simulink model "SingleTrack"  (Simulink 10.3)
settings: Solver=ode45  StartTime=0.0  StopTime=inf  FixedStep=0.001  RelTol=1e-3
PreLoadFcn:
  | SingleTrack_params
undefined symbols (not defined in the file or in its folder): Car_Bdy1_mass, Car_Steering_i, Car_Whl_Radius, Car_WhlBaseF, Car_WhlBaseR, mEngineMax, PT_DL_iDiff, PT_GearBox_iForwardGears
libraries: CarMaker4SL x9
(part 4 of 4)

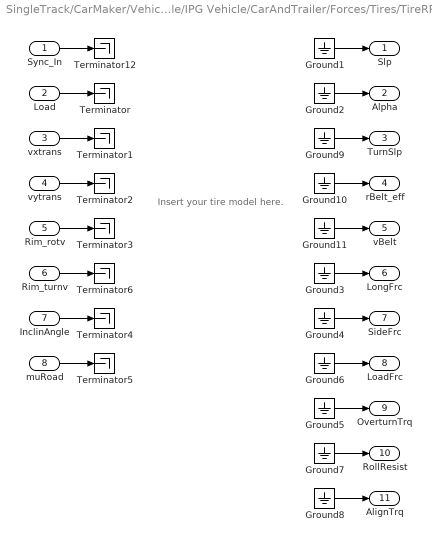
== system SingleTrack/CarMaker/Vehicle/IPG Vehicle/CarAndTrailer/Forces/Tires/TireRR ==
  note: Insert your tire model here.
  Sync_In : Inport
  Load : Inport  Port=2
  vxtrans : Inport  Port=3
  vytrans : Inport  Port=4
  Rim_rotv : Inport  Port=5
  Rim_turnv : Inport  Port=6
  InclinAngle : Inport  Port=7
  muRoad : Inport  Port=8
  Ground{1..11} (11 alike) : Ground
  Terminator{,1..6,12} (8 alike) : Terminator
  Slp : Outport  VectorParamsAs1DForOutWhenUnconnected=off
  Alpha : Outport  Port=2  VectorParamsAs1DForOutWhenUnconnected=off
  TurnSlp : Outport  Port=3  VectorParamsAs1DForOutWhenUnconnected=off
  rBelt_eff : Outport  Port=4  VectorParamsAs1DForOutWhenUnconnected=off
  vBelt : Outport  Port=5  VectorParamsAs1DForOutWhenUnconnected=off
  LongFrc : Outport  Port=6  VectorParamsAs1DForOutWhenUnconnected=off
  SideFrc : Outport  Port=7  VectorParamsAs1DForOutWhenUnconnected=off
  LoadFrc : Outport  Port=8  VectorParamsAs1DForOutWhenUnconnected=off
  OverturnTrq : Outport  Port=9  VectorParamsAs1DForOutWhenUnconnected=off
  RollResist : Outport  Port=10  VectorParamsAs1DForOutWhenUnconnected=off
  AlignTrq : Outport  Port=11  VectorParamsAs1DForOutWhenUnconnected=off
  wires:
  Ground11/1 -> vBelt/1
  Ground10/1 -> rBelt_eff/1
  Ground9/1 -> TurnSlp/1
  Rim_turnv/1 -> Terminator6/1
  Sync_In/1 -> Terminator12/1
  Ground2/1 -> Alpha/1
  Ground3/1 -> LongFrc/1
  Ground4/1 -> SideFrc/1
  Ground5/1 -> OverturnTrq/1
  vxtrans/1 -> Terminator1/1
  vytrans/1 -> Terminator2/1
  Rim_rotv/1 -> Terminator3/1
  InclinAngle/1 -> Terminator4/1
  muRoad/1 -> Terminator5/1
  Load/1 -> Terminator/1
  Ground1/1 -> Slp/1
  Ground6/1 -> LoadFrc/1
  Ground7/1 -> RollResist/1
  Ground8/1 -> AlignTrq/1

== system SingleTrack/CarMaker/Vehicle/User Vehicle (CM4SL)/CarAndTrailer/CreateBus Vhcl.Fr1/Tr2Fr0/Subsystem_00 ==
  sincos : Inport
  Bus Selector : BusSelector  OutputSignals=cry,crz
  Product : Product  RndMeth=Zero
  Tr2Fr1_00 : Outport  VectorParamsAs1DForOutWhenUnconnected=off
  wires:
  sincos/1 -> Bus Selector/1
  Product/1 -> Tr2Fr1_00/1
  Bus Selector/1 -> Product/1  "<cry>"
  Bus Selector/2 -> Product/2  "<crz>"

== system SingleTrack/CarMaker/Vehicle/User Vehicle (CM4SL)/CarAndTrailer/CreateBus Vhcl.Fr1/Tr2Fr0/Subsystem_01 ==
  sincos : Inport
  Add : Sum  Inputs=+-
  Bus Selector : BusSelector  OutputSignals=srx,sry,crz,crx,srz
  Product : Product  Inputs=3  RndMeth=Zero
  Product1 : Product  RndMeth=Zero
  Tr2Fr1_01 : Outport  VectorParamsAs1DForOutWhenUnconnected=off
  wires:
  sincos/1 -> Bus Selector/1
  Product/1 -> Add/1
  Product1/1 -> Add/2
  Add/1 -> Tr2Fr1_01/1
  Bus Selector/1 -> Product/1  "<srx>"
  Bus Selector/2 -> Product/2  "<sry>"
  Bus Selector/3 -> Product/3  "<crz>"
  Bus Selector/4 -> Product1/1  "<crx>"
  Bus Selector/5 -> Product1/2  "<srz>"

== system SingleTrack/CarMaker/Vehicle/User Vehicle (CM4SL)/CarAndTrailer/CreateBus Vhcl.Fr1/Tr2Fr0/Subsystem_02 ==
  sincos : Inport
  Add : Sum
  Bus Selector : BusSelector  OutputSignals=crx,sry,crz,srx,srz
  Product : Product  Inputs=3  RndMeth=Zero
  Product1 : Product  RndMeth=Zero
  Tr2Fr1_02 : Outport  VectorParamsAs1DForOutWhenUnconnected=off
  wires:
  Add/1 -> Tr2Fr1_02/1
  Product1/1 -> Add/2
  Product/1 -> Add/1
  sincos/1 -> Bus Selector/1
  Bus Selector/1 -> Product/1  "<crx>"
  Bus Selector/2 -> Product/2  "<sry>"
  Bus Selector/3 -> Product/3  "<crz>"
  Bus Selector/5 -> Product1/2  "<srz>"
  Bus Selector/4 -> Product1/1  "<srx>"

== system SingleTrack/CarMaker/Vehicle/User Vehicle (CM4SL)/CarAndTrailer/CreateBus Vhcl.Fr1/Tr2Fr0/Subsystem_10 ==
  sincos : Inport
  Bus Selector : BusSelector  OutputSignals=cry,srz
  Product : Product  RndMeth=Zero
  Tr2Fr1_10 : Outport  VectorParamsAs1DForOutWhenUnconnected=off
  wires:
  Bus Selector/2 -> Product/2  "<srz>"
  Bus Selector/1 -> Product/1  "<cry>"
  Product/1 -> Tr2Fr1_10/1
  sincos/1 -> Bus Selector/1

== system SingleTrack/CarMaker/Vehicle/User Vehicle (CM4SL)/CarAndTrailer/CreateBus Vhcl.Fr1/Tr2Fr0/Subsystem_11 ==
  sincos : Inport
  Add : Sum
  Bus Selector : BusSelector  OutputSignals=srx,sry,srz,crx,crz
  Product : Product  Inputs=3  RndMeth=Zero
  Product1 : Product  RndMeth=Zero
  Tr2Fr1_11 : Outport  VectorParamsAs1DForOutWhenUnconnected=off
  wires:
  sincos/1 -> Bus Selector/1
  Product/1 -> Add/1
  Product1/1 -> Add/2
  Add/1 -> Tr2Fr1_11/1
  Bus Selector/1 -> Product/1  "<srx>"
  Bus Selector/2 -> Product/2  "<sry>"
  Bus Selector/3 -> Product/3  "<srz>"
  Bus Selector/5 -> Product1/2  "<crz>"
  Bus Selector/4 -> Product1/1  "<crx>"

== system SingleTrack/CarMaker/Vehicle/User Vehicle (CM4SL)/CarAndTrailer/CreateBus Vhcl.Fr1/Tr2Fr0/Subsystem_12 ==
  sincos : Inport
  Add : Sum  Inputs=+-
  Bus Selector : BusSelector  OutputSignals=crx,sry,srz,srx,crz
  Product : Product  Inputs=3  RndMeth=Zero
  Product1 : Product  RndMeth=Zero
  Tr2Fr1_12 : Outport  VectorParamsAs1DForOutWhenUnconnected=off
  wires:
  Add/1 -> Tr2Fr1_12/1
  Product1/1 -> Add/2
  Product/1 -> Add/1
  sincos/1 -> Bus Selector/1
  Bus Selector/1 -> Product/1  "<crx>"
  Bus Selector/2 -> Product/2  "<sry>"
  Bus Selector/3 -> Product/3  "<srz>"
  Bus Selector/5 -> Product1/2  "<crz>"
  Bus Selector/4 -> Product1/1  "<srx>"

== system SingleTrack/CarMaker/Vehicle/User Vehicle (CM4SL)/CarAndTrailer/CreateBus Vhcl.Fr1/Tr2Fr0/Subsystem_20 ==
  sincos : Inport
  Bus Selector : BusSelector  OutputSignals=sry
  Gain : Gain  Gain=-1
  Tr2Fr1_20 : Outport  VectorParamsAs1DForOutWhenUnconnected=off
  wires:
  sincos/1 -> Bus Selector/1
  Gain/1 -> Tr2Fr1_20/1
  Bus Selector/1 -> Gain/1  "<sry>"

== system SingleTrack/CarMaker/Vehicle/User Vehicle (CM4SL)/CarAndTrailer/CreateBus Vhcl.Fr1/Tr2Fr0/Subsystem_21 ==
  sincos : Inport
  Bus Selector : BusSelector  OutputSignals=srx,cry
  Product : Product  RndMeth=Zero
  Tr2Fr1_21 : Outport  VectorParamsAs1DForOutWhenUnconnected=off
  wires:
  sincos/1 -> Bus Selector/1
  Product/1 -> Tr2Fr1_21/1
  Bus Selector/1 -> Product/1  "<srx>"
  Bus Selector/2 -> Product/2  "<cry>"

== system SingleTrack/CarMaker/Vehicle/User Vehicle (CM4SL)/CarAndTrailer/CreateBus Vhcl.Fr1/Tr2Fr0/Subsystem_22 ==
  sincos : Inport
  Bus Selector : BusSelector  OutputSignals=crx,cry
  Product : Product  RndMeth=Zero
  Tr2Fr1_22 : Outport  VectorParamsAs1DForOutWhenUnconnected=off
  wires:
  Product/1 -> Tr2Fr1_22/1
  sincos/1 -> Bus Selector/1
  Bus Selector/1 -> Product/1  "<crx>"
  Bus Selector/2 -> Product/2  "<cry>"

== system SingleTrack/CarMaker/Vehicle/User Vehicle (CM4SL)/CarAndTrailer/CreateBus Vhcl.Fr1/Tr2Fr0/sincos ==
  Car : Inport
  Bus Creator : BusCreator  Inputs=6
  Bus Selector : BusSelector  OutputSignals=Road_Fr1_rx,Road_Fr1_ry,Car_Yaw
  Trigonometric Function : Trigonometry
  Trigonometric Function1 : Trigonometry  Operator=cos
  Trigonometric Function2 : Trigonometry
  Trigonometric Function3 : Trigonometry
  Trigonometric Function4 : Trigonometry  Operator=cos
  Trigonometric Function5 : Trigonometry  Operator=cos
  sincos : Outport  VectorParamsAs1DForOutWhenUnconnected=off
  wires:
  Bus Selector/1 -> Trigonometric Function/1, Trigonometric Function1/1  "<Road_Fr1_rx>"
  Bus Selector/2 -> Trigonometric Function3/1, Trigonometric Function4/1  "<Road_Fr1_ry>"
  Bus Selector/3 -> Trigonometric Function2/1, Trigonometric Function5/1  "<Car_Yaw>"
  Car/1 -> Bus Selector/1
  Trigonometric Function5/1 -> Bus Creator/6  "crz"
  Trigonometric Function4/1 -> Bus Creator/5  "cry"
  Trigonometric Function1/1 -> Bus Creator/4  "crx"
  Trigonometric Function2/1 -> Bus Creator/3  "srz"
  Trigonometric Function3/1 -> Bus Creator/2  "sry"
  Trigonometric Function/1 -> Bus Creator/1  "srx"
  Bus Creator/1 -> sincos/1

== system SingleTrack/CarMaker/Vehicle/User Vehicle (CM4SL)/CarAndTrailer/PowerTrainUpd/Set OperationState/If Action Subsystem ==
  note: If steering wheel angle is zero, OperationState equals to the desired State by VhclOperator,
  note: else the last value is kept.
  In1 : Inport
  Action Port : ActionPort  ActionPortLabel=if { }
  Abs : Abs
  If : If  IfExpression=u1 <= 0.0175
  If Action Subsystem : Subsystem  TreatAsAtomicUnit=on
  If Action Subsystem1 : Subsystem  TreatAsAtomicUnit=on
  Merge : Merge
  Read CM Dict1 : CarMaker4SL/Read CM Dict  xname=VC.Steer.Ang  xsync=off  xstime=Continuous
  Read CM Dict2 : CarMaker4SL/Read CM Dict  xname=Vhcl.OperationState  xsync=off  xstime=Continuous
  Out1 : Outport  VectorParamsAs1DForOutWhenUnconnected=off
  wires:
  Read CM Dict1/1 -> Abs/1
  Abs/1 -> If/1
  If/1 -> If Action Subsystem/Action
  Merge/1 -> Out1/1
  If Action Subsystem/1(Out1) -> Merge/1
  In1/1 -> If Action Subsystem/1(In1)
  If Action Subsystem1/1(Out1) -> Merge/2
  If/2 -> If Action Subsystem1/Action
  Read CM Dict2/1 -> If Action Subsystem1/1(In1)

== system SingleTrack/CarMaker/Vehicle/User Vehicle (CM4SL)/CarAndTrailer/PowerTrainUpd/Set OperationState/If Action Subsystem1 ==
  In1 : Inport
  Action Port : ActionPort  ActionPortLabel=else { }
  Out1 : Outport  VectorParamsAs1DForOutWhenUnconnected=off
  wires:
  In1/1 -> Out1/1

== system SingleTrack/CarMaker/Vehicle/User Vehicle (CM4SL)/CarAndTrailer/single-track mass point model/Car.v_1/PassIfSim ==
  note: Output original value only when simulating,
      | and zero during pre- or postprocessing.
  In1 : Inport
  "   " : Product  InputSameDT=on  SaturateOnIntegerOverflow=on  OutDataTypeStr=Inherit: Same as first input
  Data Type Conversion : DataTypeConversion
  Out1 : Outport  VectorParamsAs1DForOutWhenUnconnected=off
  wires:
  [TRSim] -> Data Type Conversion/1
  "   "/1 -> Out1/1
  Data Type Conversion/1 -> "   "/2
  In1/1 -> "   "/1

== system SingleTrack/CarMaker/Vehicle/User Vehicle (CM4SL)/CarAndTrailer/single-track mass point model/Vehicle Initial Cfg/CreateBus Vhcl.Cfg ==
  In1 : Inport
  Bus Creator : BusCreator  Inputs=13
  Demux : Demux  Outputs=13
      settings: DisplayOption=none
  Out1 : Outport  VectorParamsAs1DForOutWhenUnconnected=off
  wires:
  Demux/13 -> Bus Creator/13  "Vhcl Cfg Whl_rotv RR"
  Bus Creator/1 -> Out1/1
  In1/1 -> Demux/1
  Demux/12 -> Bus Creator/12  "Vhcl Cfg Whl_rotv RL"
  Demux/11 -> Bus Creator/11  "Vhcl Cfg Whl_rotv FR"
  Demux/10 -> Bus Creator/10  "Vhcl Cfg Whl_rotv FL"
  Demux/9 -> Bus Creator/9  "SimCore Trailer nTrailers"
  Demux/8 -> Bus Creator/8  "Vhcl Cfg GearBox_rotv_out"
  Demux/7 -> Bus Creator/7  "Vhcl Cfg Engine_rotv"
  Demux/6 -> Bus Creator/6  "Vhcl Cfg Pitch"
  Demux/5 -> Bus Creator/5  "Vhcl Cfg Yaw"
  Demux/4 -> Bus Creator/4  "Vhcl Cfg Roll"
  Demux/2 -> Bus Creator/2  "Vhcl Cfg Fr1_Pos y"
  Demux/1 -> Bus Creator/1  "Vhcl Cfg Fr1_Pos x"
  Demux/3 -> Bus Creator/3  "Vhcl Cfg Fr1_Pos z"

== system SingleTrack/CarMaker/Vehicle/User Vehicle (CM4SL)/CarAndTrailer/single-track mass point model/yaw/Vehicle Initial Cfg ==
  CreateBus Vhcl.Cfg : Subsystem
  VehicleControlUpd : S-Function  FunctionName=cm_initial  SFunctionDeploymentMode=off  EnableBusSupport=off
  Vhcl.Cfg : Outport  VectorParamsAs1DForOutWhenUnconnected=off
  wires:
  VehicleControlUpd/1 -> CreateBus Vhcl.Cfg/1(In1)
  CreateBus Vhcl.Cfg/1(Out1) -> Vhcl.Cfg/1

== system SingleTrack/CarMaker/Vehicle/User Vehicle (CM4SL)/CarAndTrailer/single-track mass point model/yaw/side forces ==
  vYaw : Inport
  beta : Inport  Port=2
  v : Inport  Port=3
  StWhlAngle : Inport  Port=4
  " " : Product  InputSameDT=on  SaturateOnIntegerOverflow=on  OutDataTypeStr=Inherit: Same as first input
  "  " : Product  InputSameDT=on  SaturateOnIntegerOverflow=on  OutDataTypeStr=Inherit: Same as first input
  "            " : Product  InputSameDT=on  SaturateOnIntegerOverflow=on  OutDataTypeStr=Inherit: Same as first input
  "S_R * l_R " : Product  InputSameDT=on  SaturateOnIntegerOverflow=on  OutDataTypeStr=Inherit: Same as first input
  "S_V * l_V " : Product  InputSameDT=on  SaturateOnIntegerOverflow=on  OutDataTypeStr=Inherit: Same as first input
  Subsystem : Subsystem
  Sum : Sum  InputSameDT=on  SaturateOnIntegerOverflow=on  OutDataTypeStr=Inherit: Same as first input
  Sum1 : Sum  Inputs=-+  InputSameDT=on  SaturateOnIntegerOverflow=on  OutDataTypeStr=Inherit: Same as first input
  Sum4 : Sum  Inputs=+-  InputSameDT=on  SaturateOnIntegerOverflow=on  OutDataTypeStr=Inherit: Same as first input
  c_alphaR : Gain  Gain=50000  SaturateOnIntegerOverflow=on  OutDataTypeStr=Inherit: Same as input  ParamDataTypeStr=Inherit: Same as input
  front wheel steering lock angle : Subsystem
  l__F : Constant  Value=Car_WhlBaseF
  l__R : Constant  Value=-Car_WhlBaseR
  S_F * l_F : Outport  VectorParamsAs1DForOutWhenUnconnected=off
  S_R * l_R : Outport  Port=2  VectorParamsAs1DForOutWhenUnconnected=off
  S_V : Outport  Port=3  VectorParamsAs1DForOutWhenUnconnected=off
  S_R : Outport  Port=4  VectorParamsAs1DForOutWhenUnconnected=off
  alpha_F : Outport  Port=5  VectorParamsAs1DForOutWhenUnconnected=off
  alpha_R : Outport  Port=6  VectorParamsAs1DForOutWhenUnconnected=off
  wires:
  front wheel steering lock angle/1(c_alphaF) -> "            "/1
  StWhlAngle/1 -> front wheel steering lock angle/1(StWhlAngle)
  "S_R * l_R "/1 -> S_R * l_R/1
  Sum4/1 -> alpha_F/1, "            "/2
  front wheel steering lock angle/2(delta_F) -> Sum4/1
  Sum/1 -> front wheel steering lock angle/2(beta + l_F * vYaw / v), Sum4/2
  v/1 -> Subsystem/1(v)
  vYaw/1 -> Subsystem/2(vYaw)
  "S_V * l_V "/1 -> S_F * l_F/1
  "            "/1 -> S_V/1, "S_V * l_V "/1
  c_alphaR/1 -> S_R/1, "S_R * l_R "/1
  Sum1/1 -> alpha_R/1, c_alphaR/1
  "  "/1 -> Sum/2
  " "/1 -> Sum1/2
  l__R/1 -> "S_R * l_R "/2, " "/2
  Subsystem/1(vYaw/v) -> "  "/2, " "/1
  l__F/1 -> "S_V * l_V "/2, "  "/1
  beta/1 -> Sum/1, Sum1/1

== system SingleTrack/CarMaker/Vehicle/User Vehicle (CM4SL)/CarAndTrailer/single-track mass point model/yaw/sideslip angle ==
  vYaw : Inport
  m : Inport  Port=2
  v_dot : Inport  Port=3
  v : Inport  Port=4
  S : Inport  Port=5
  " " : Product  Inputs=*/  InputSameDT=on  SaturateOnIntegerOverflow=on  OutDataTypeStr=Inherit: Same as first input
  "  " : Product  InputSameDT=on  SaturateOnIntegerOverflow=on  OutDataTypeStr=Inherit: Same as first input
  Subsystem : Subsystem
  Sum2 : Sum  Inputs=+-  InputSameDT=on  SaturateOnIntegerOverflow=on  OutDataTypeStr=Inherit: Same as first input
  beta_dot * dt : Integrator  ExternalReset=level
  beta_dot : Outport  VectorParamsAs1DForOutWhenUnconnected=off
  beta : Outport  Port=2  VectorParamsAs1DForOutWhenUnconnected=off
  wires:
  v/1 -> Subsystem/2(v)
  Subsystem/1(Out1) -> beta_dot/1, beta_dot * dt/1
  vYaw/1 -> Subsystem/1(vYaw)
  Sum2/1 -> Subsystem/3(In3)
  "  "/1 -> Sum2/2
  m/1 -> " "/2
  v_dot/1 -> "  "/1
  " "/1 -> Sum2/1
  S/1 -> " "/1
  beta_dot * dt/1 -> "  "/2, beta/1
  [TRStart] -> beta_dot * dt/2

== system SingleTrack/CarMaker/Vehicle/User Vehicle (CM4SL)/CarAndTrailer/PowerTrainUpd/Set OperationState/If Action Subsystem/If Action Subsystem ==
  In1 : Inport
  Action Port : ActionPort  ActionPortLabel=if { }
  Out1 : Outport  VectorParamsAs1DForOutWhenUnconnected=off
  wires:
  In1/1 -> Out1/1

== system SingleTrack/CarMaker/Vehicle/User Vehicle (CM4SL)/CarAndTrailer/PowerTrainUpd/Set OperationState/If Action Subsystem/If Action Subsystem1 ==
  In1 : Inport
  Action Port : ActionPort  ActionPortLabel=else { }
  Out1 : Outport  VectorParamsAs1DForOutWhenUnconnected=off
  wires:
  In1/1 -> Out1/1

== system SingleTrack/CarMaker/Vehicle/User Vehicle (CM4SL)/CarAndTrailer/single-track mass point model/yaw/Vehicle Initial Cfg/CreateBus Vhcl.Cfg ==
  In1 : Inport
  Bus Creator : BusCreator  Inputs=13
  Demux : Demux  Outputs=13
      settings: DisplayOption=none
  Out1 : Outport  VectorParamsAs1DForOutWhenUnconnected=off
  wires:
  Demux/13 -> Bus Creator/13  "Vhcl Cfg Whl_rotv RR"
  Bus Creator/1 -> Out1/1
  In1/1 -> Demux/1
  Demux/12 -> Bus Creator/12  "Vhcl Cfg Whl_rotv RL"
  Demux/11 -> Bus Creator/11  "Vhcl Cfg Whl_rotv FR"
  Demux/10 -> Bus Creator/10  "Vhcl Cfg Whl_rotv FL"
  Demux/9 -> Bus Creator/9  "SimCore Trailer nTrailers"
  Demux/8 -> Bus Creator/8  "Vhcl Cfg GearBox_rotv_out"
  Demux/7 -> Bus Creator/7  "Vhcl Cfg Engine_rotv"
  Demux/6 -> Bus Creator/6  "Vhcl Cfg Pitch"
  Demux/5 -> Bus Creator/5  "Vhcl Cfg Yaw"
  Demux/4 -> Bus Creator/4  "Vhcl Cfg Roll"
  Demux/2 -> Bus Creator/2  "Vhcl Cfg Fr1_Pos y"
  Demux/1 -> Bus Creator/1  "Vhcl Cfg Fr1_Pos x"
  Demux/3 -> Bus Creator/3  "Vhcl Cfg Fr1_Pos z"

== system SingleTrack/CarMaker/Vehicle/User Vehicle (CM4SL)/CarAndTrailer/single-track mass point model/yaw/side forces/Subsystem ==
  v : Inport
  vYaw : Inport  Port=2
  If : If  IfExpression=u1 > 0.1 | u1 < -0.1
  If Action Subsystem : Subsystem  TreatAsAtomicUnit=on
  If Action Subsystem1 : Subsystem  TreatAsAtomicUnit=on
  Merge : Merge  InitialOutput=0
  vYaw/v : Outport  VectorParamsAs1DForOutWhenUnconnected=off
  wires:
  v/1 -> If Action Subsystem/1(v), If/1
  vYaw/1 -> If Action Subsystem/2(vYaw)
  If/1 -> If Action Subsystem/Action
  If/2 -> If Action Subsystem1/Action
  Merge/1 -> vYaw/v/1
  If Action Subsystem/1(Out1) -> Merge/1
  If Action Subsystem1/1(Out1) -> Merge/2

== system SingleTrack/CarMaker/Vehicle/User Vehicle (CM4SL)/CarAndTrailer/single-track mass point model/yaw/side forces/front wheel steering lock angle ==
  StWhlAngle : Inport
  beta + l_F * vYaw / v : Inport  Port=2
  "   " : Product  InputSameDT=on  SaturateOnIntegerOverflow=on  OutDataTypeStr=Inherit: Same as first input
  "     " : Constant
  "      " : Product  Inputs=*/  InputSameDT=on  SaturateOnIntegerOverflow=on  OutDataTypeStr=Inherit: Same as first input
  "       " : Product  Inputs=*/*  InputSameDT=on  SaturateOnIntegerOverflow=on  OutDataTypeStr=Inherit: Same as first input
  1/ i_S : Gain  Gain=1/Car_Steering_i  SaturateOnIntegerOverflow=on  OutDataTypeStr=Inherit: Same as input  ParamDataTypeStr=Inherit: Same as input
  C_S : Constant  Value=10000
  Sum2 : Sum  InputSameDT=on  SaturateOnIntegerOverflow=on  OutDataTypeStr=Inherit: Same as first input
  Sum3 : Sum  InputSameDT=on  SaturateOnIntegerOverflow=on  OutDataTypeStr=Inherit: Same as first input
  "c_alphaF " : Constant  Value=50000
  n_F : Constant  Value=0.06
  c_alphaF : Outport  VectorParamsAs1DForOutWhenUnconnected=off
  delta_F : Outport  Port=2  VectorParamsAs1DForOutWhenUnconnected=off
  wires:
  "      "/1 -> delta_F/1
  "c_alphaF "/1 -> "       "/1, c_alphaF/1
  n_F/1 -> "       "/3
  C_S/1 -> "       "/2
  Sum2/1 -> "      "/1
  Sum3/1 -> "      "/2
  "     "/1 -> Sum3/1
  1/ i_S/1 -> Sum2/1
  "   "/1 -> Sum2/2
  StWhlAngle/1 -> 1/ i_S/1
  "       "/1 -> "   "/1, Sum3/2
  beta + l_F * vYaw / v/1 -> "   "/2

== system SingleTrack/CarMaker/Vehicle/User Vehicle (CM4SL)/CarAndTrailer/single-track mass point model/yaw/sideslip angle/Subsystem ==
  vYaw : Inport
  v : Inport  Port=2
  In3 : Inport  Port=3
  If : If  IfExpression=u1 > 0.1 | u1 < -0.1
  If Action Subsystem : Subsystem  TreatAsAtomicUnit=on
  If Action Subsystem1 : Subsystem  TreatAsAtomicUnit=on
  Merge : Merge
  Sum1 : Sum  Inputs=-+  InputSameDT=on  SaturateOnIntegerOverflow=on  OutDataTypeStr=Inherit: Same as first input
  Out1 : Outport  VectorParamsAs1DForOutWhenUnconnected=off
  wires:
  vYaw/1 -> Sum1/1
  v/1 -> If Action Subsystem/1(v), If/1
  Sum1/1 -> Out1/1
  If Action Subsystem/1(Out1) -> Merge/1
  If Action Subsystem1/1(Out1) -> Merge/2
  Merge/1 -> Sum1/2
  If/2 -> If Action Subsystem1/Action
  In3/1 -> If Action Subsystem/2(In3)
  If/1 -> If Action Subsystem/Action

== system SingleTrack/CarMaker/Vehicle/User Vehicle (CM4SL)/CarAndTrailer/single-track mass point model/yaw/side forces/Subsystem/If Action Subsystem ==
  v : Inport
  vYaw : Inport  Port=2
  Action Port : ActionPort  ActionPortLabel=if { }
  vYaw / v : Product  Inputs=/*  InputSameDT=on  SaturateOnIntegerOverflow=on  OutDataTypeStr=Inherit: Same as first input
  Out1 : Outport  InitialOutput=0  VectorParamsAs1DForOutWhenUnconnected=off
  wires:
  v/1 -> vYaw / v/1
  vYaw/1 -> vYaw / v/2
  vYaw / v/1 -> Out1/1

== system SingleTrack/CarMaker/Vehicle/User Vehicle (CM4SL)/CarAndTrailer/single-track mass point model/yaw/side forces/Subsystem/If Action Subsystem1 ==
  Action Port : ActionPort  ActionPortLabel=else { }
  Constant : Constant  Value=0
  Out1 : Outport  InitialOutput=0  VectorParamsAs1DForOutWhenUnconnected=off
  wires:
  Constant/1 -> Out1/1

== system SingleTrack/CarMaker/Vehicle/User Vehicle (CM4SL)/CarAndTrailer/single-track mass point model/yaw/sideslip angle/Subsystem/If Action Subsystem ==
  v : Inport
  In3 : Inport  Port=2
  Action Port : ActionPort  ActionPortLabel=if { }
  "    " : Product  Inputs=/*  InputSameDT=on  SaturateOnIntegerOverflow=on  OutDataTypeStr=Inherit: Same as first input
  Out1 : Outport  InitialOutput=0  VectorParamsAs1DForOutWhenUnconnected=off
  wires:
  v/1 -> "    "/1
  In3/1 -> "    "/2
  "    "/1 -> Out1/1

== system SingleTrack/CarMaker/Vehicle/User Vehicle (CM4SL)/CarAndTrailer/single-track mass point model/yaw/sideslip angle/Subsystem/If Action Subsystem1 ==
  Action Port : ActionPort  ActionPortLabel=else { }
  Constant : Constant  Value=0
  Out1 : Outport  InitialOutput=0  VectorParamsAs1DForOutWhenUnconnected=off
  wires:
  Constant/1 -> Out1/1
